simulink model "week3"  (R2024b)
settings: Solver=ode4  StartTime=0.0  StopTime=10.0  FixedStep=0.001  RelTol=1e-3
values from neighbouring files (symbols this model uses):
  c1 = 350    [Project.m]
  c2 = 15000    [Project.m]
  k1 = 80000    [Project.m]
  k2 = 500000    [Project.m]
  m1 = 2500    [Project.m]
  m2 = 320    [Project.m]
settings Model: Creator=elija  LastModifiedBy=elija

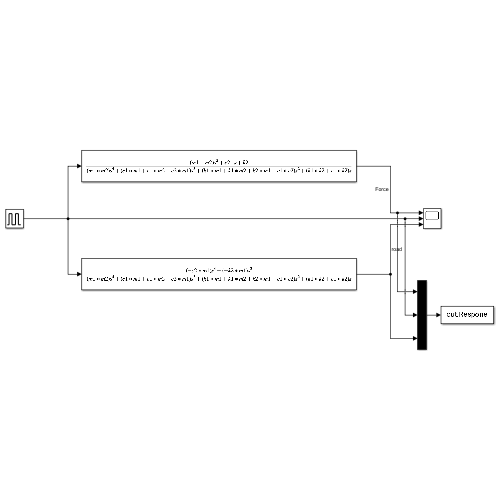
[thumbnail: Simulink's stored preview of the top-level diagram]
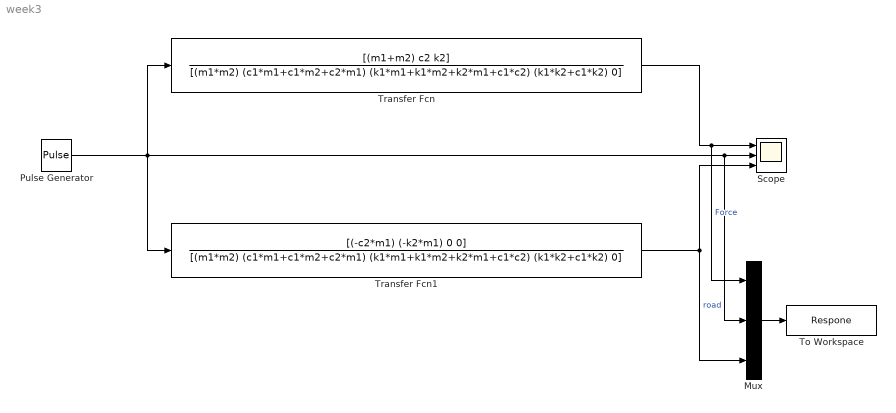
== system week3 ==
  Mux : Mux  Inputs=3
  Pulse Generator : DiscretePulseGenerator  PulseType=Time based  Period=10  PulseWidth=50  PhaseDelay=2
  Scope : Scope  NumInputPorts=3
  To Workspace : ToWorkspace  VariableName=Respone  SaveFormat=Timeseries  SampleTime=-1
  Transfer Fcn : TransferFcn  Numerator=[(m1+m2) c2 k2]  Denominator=[(m1*m2) (c1*m1+c1*m2+c2*m1) (k1*m1+k1*m2+k2*m1+c1*c2) (k1*k2+c1*k2) 0]
  Transfer Fcn1 : TransferFcn  Numerator=[(-c2*m1) (-k2*m1) 0 0]  Denominator=[(m1*m2) (c1*m1+c1*m2+c2*m1) (k1*m1+k1*m2+k2*m1+c1*c2) (k1*k2+c1*k2) 0]
  wires:
  Pulse Generator/1 -> Transfer Fcn1/1, Transfer Fcn/1, Mux/2, Scope/2
  Transfer Fcn/1 -> Mux/1, Scope/1  "Force"
  Transfer Fcn1/1 -> Scope/3, Mux/3  "road"
  Mux/1 -> To Workspace/1
